simulink model "ASLquad_onboardRobustMPC_mdl"  (Simulink 8.1)
settings: Solver=ode45  StartTime=0.0  StopTime=10.0  RelTol=1e-3
values from neighbouring files (symbols this model uses):
  ASLquad_RobustMPC =     [ASLquad_RobustMPC_v2x.mat]    (also in ASLquad_RobustMPC_v3_x_Nfour.mat; ASLquad_RobustMPC_v3xyz.mat; ASLquad_RobustMPC_v3xyz_v2.mat; ASLquad_RobustMPC_v3xz.mat)
libraries: Robust_MPC_Library x6
settings Model: Creator=Kostas  LastModifiedBy=Kostas
settings DataIOCC: SignalLoggingSaveFormat=Dataset
settings OptimizationCC: ExpressionDepthLimit=128
settings DebuggingCC: FcnCallInpInsideContextMsg=EnableAllAsError
settings GRTTargetCC: CombineOutputUpdateFcns=on  GRTInterface=off

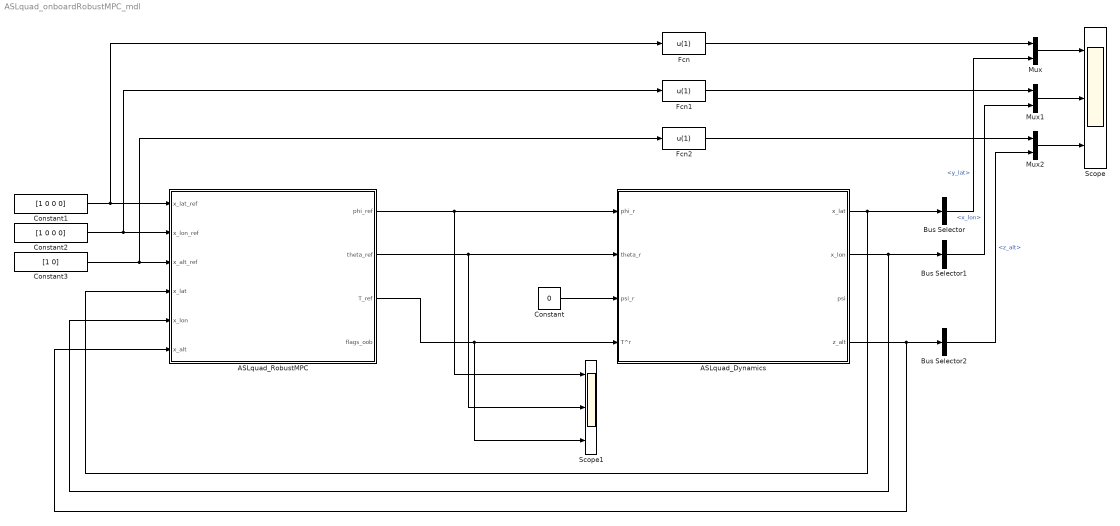
== system ASLquad_onboardRobustMPC_mdl ==
  ASLquad_Dynamics : Subsystem
  ASLquad_RobustMPC : Subsystem
  Bus Selector : BusSelector  OutputSignals=y_lat
  Bus Selector1 : BusSelector  OutputSignals=x_lon
  Bus Selector2 : BusSelector  OutputSignals=z_alt
  Constant : Constant  Value=0
  Constant1 : Constant  Value=[1 0 0 0]
  Constant2 : Constant  Value=[1 0 0 0]
  Constant3 : Constant  Value=[1 0]
  Fcn : Fcn  Expr=u(1)
  Fcn1 : Fcn  Expr=u(1)
  Fcn2 : Fcn  Expr=u(1)
  Mux : Mux  Inputs=2
  Mux1 : Mux  Inputs=2
  Mux2 : Mux  Inputs=2
  Scope : Scope  NumInputPorts=3
      settings: YMin=0.9995~-5~-5  YMax=1.00525~5~5
  Scope1 : Scope  NumInputPorts=3
      settings: YMin=-25~-5~-5  YMax=325~5~5
  wires:
  ASLquad_RobustMPC/1(phi_ref) -> Scope1/1, ASLquad_Dynamics/1(phi_r)
  ASLquad_RobustMPC/2(theta_ref) -> Scope1/2, ASLquad_Dynamics/2(theta_r)
  ASLquad_RobustMPC/3(T_ref) -> Scope1/3, ASLquad_Dynamics/4(T^r)
  Constant/1 -> ASLquad_Dynamics/3(psi_r)
  ASLquad_Dynamics/1(x_lat) -> Bus Selector/1, ASLquad_RobustMPC/4(x_lat)
  ASLquad_Dynamics/2(x_lon) -> Bus Selector1/1, ASLquad_RobustMPC/5(x_lon)
  ASLquad_Dynamics/4(z_alt) -> Bus Selector2/1, ASLquad_RobustMPC/6(x_alt)
  Constant2/1 -> Fcn1/1, ASLquad_RobustMPC/2(x_lon_ref)
  Constant3/1 -> Fcn2/1, ASLquad_RobustMPC/3(x_alt_ref)
  Constant1/1 -> Fcn/1, ASLquad_RobustMPC/1(x_lat_ref)
  Fcn/1 -> Mux/1
  Fcn1/1 -> Mux1/1
  Fcn2/1 -> Mux2/1
  Bus Selector/1 -> Mux/2  "<y_lat>"
  Bus Selector1/1 -> Mux1/2  "<x_lon>"
  Bus Selector2/1 -> Mux2/2  "<z_alt>"
  Mux/1 -> Scope/1
  Mux1/1 -> Scope/2
  Mux2/1 -> Scope/3

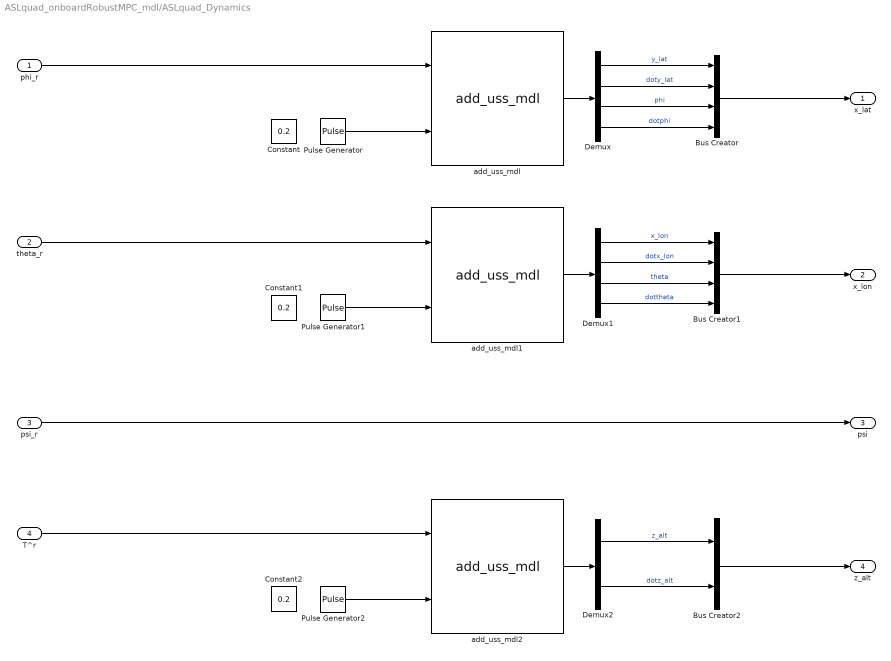
== system ASLquad_onboardRobustMPC_mdl/ASLquad_Dynamics ==
  phi_r : Inport
  theta_r : Inport  Port=2
  psi_r : Inport  Port=3
  T^r : Inport  Port=4
  Bus Creator : BusCreator
  Bus Creator1 : BusCreator
  Bus Creator2 : BusCreator  Inputs=2
  Constant : Constant  Value=0.2
  Constant1 : Constant  Value=0.2
  Constant2 : Constant  Value=0.2
  Demux : Demux
  Demux1 : Demux
  Demux2 : Demux  Outputs=2
  Pulse Generator : DiscretePulseGenerator  PulseType=Time based  Amplitude=.2  Period=2.5  PulseWidth=50
  Pulse Generator1 : DiscretePulseGenerator  PulseType=Time based  Amplitude=.2  Period=2.5  PulseWidth=50
  Pulse Generator2 : DiscretePulseGenerator  PulseType=Time based  Amplitude=.2  Period=2.5  PulseWidth=50
  add_uss_mdl : Robust_MPC_Library/add_uss_mdl  add_usys_d_struct=add_usys_y_d
  add_uss_mdl1 : Robust_MPC_Library/add_uss_mdl  add_usys_d_struct=add_usys_x_d
  add_uss_mdl2 : Robust_MPC_Library/add_uss_mdl  add_usys_d_struct=add_usys_z_d
  x_lat : Outport
  x_lon : Outport  Port=2
  psi : Outport  Port=3
  z_alt : Outport  Port=4
  wires:
  phi_r/1 -> add_uss_mdl/1
  theta_r/1 -> add_uss_mdl1/1
  T^r/1 -> add_uss_mdl2/1
  psi_r/1 -> psi/1
  add_uss_mdl/1 -> Demux/1
  Demux/1 -> Bus Creator/1  "y_lat"
  Demux/2 -> Bus Creator/2  "doty_lat"
  Demux/3 -> Bus Creator/3  "phi"
  Demux/4 -> Bus Creator/4  "dotphi"
  Bus Creator/1 -> x_lat/1
  add_uss_mdl1/1 -> Demux1/1
  Demux1/1 -> Bus Creator1/1  "x_lon"
  Demux1/2 -> Bus Creator1/2  "dotx_lon"
  Demux1/3 -> Bus Creator1/3  "theta"
  Demux1/4 -> Bus Creator1/4  "dottheta"
  Bus Creator1/1 -> x_lon/1
  add_uss_mdl2/1 -> Demux2/1
  Demux2/1 -> Bus Creator2/1  "z_alt"
  Demux2/2 -> Bus Creator2/2  "dotz_alt"
  Bus Creator2/1 -> z_alt/1
  Pulse Generator/1 -> add_uss_mdl/2
  Pulse Generator1/1 -> add_uss_mdl1/2
  Pulse Generator2/1 -> add_uss_mdl2/2

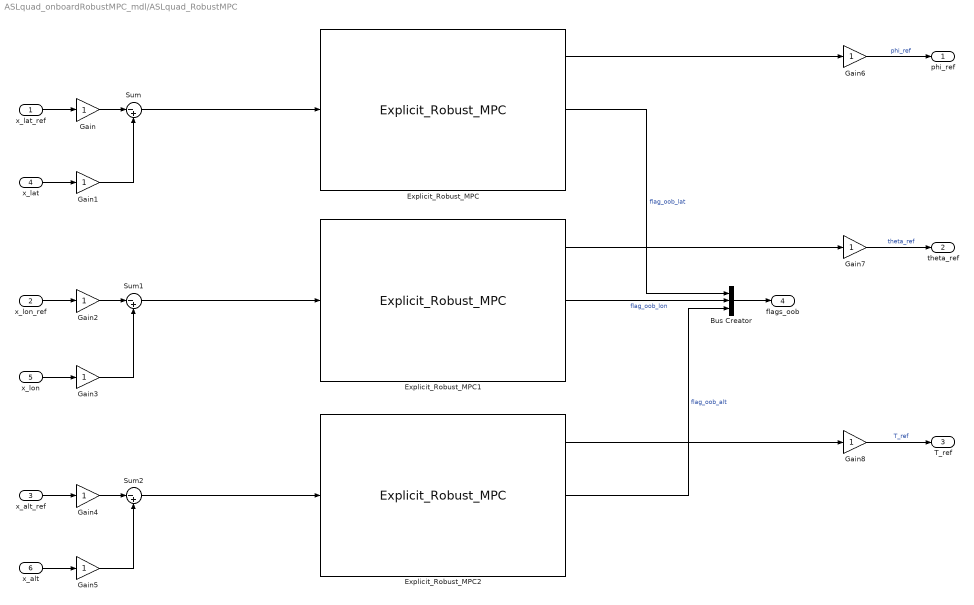
== system ASLquad_onboardRobustMPC_mdl/ASLquad_RobustMPC ==
  x_lat_ref : Inport
  x_lon_ref : Inport  Port=2
  x_alt_ref : Inport  Port=3
  x_lat : Inport  Port=4
  x_lon : Inport  Port=5
  x_alt : Inport  Port=6
  Bus Creator : BusCreator  Inputs=3
  Explicit_Robust_MPC : Robust_MPC_Library/Explicit_Robust_MPC  H=ASLquad_RobustMPC.Ydir.H  K=ASLquad_RobustMPC.Ydir.K  F=ASLquad_RobustMPC.Ydir.F  G=ASLquad_RobustMPC.Ydir.G  Nc=ASLquad_RobustMPC.Ydir.Nc  Nx=ASLquad_RobustMPC.Ydir.Nx  Hi_init=zeros(100,ASLquad_RobustMPC.Ydir.Nx)  Ki_init=zeros(100,ASLquad_RobustMPC.Ydir.Nu)
  Explicit_Robust_MPC1 : Robust_MPC_Library/Explicit_Robust_MPC  H=ASLquad_RobustMPC.Xdir.H  K=ASLquad_RobustMPC.Xdir.K  F=ASLquad_RobustMPC.Xdir.F  G=ASLquad_RobustMPC.Xdir.G  Nc=ASLquad_RobustMPC.Xdir.Nc  Nx=ASLquad_RobustMPC.Xdir.Nx  Hi_init=zeros(100,ASLquad_RobustMPC.Xdir.Nx)  Ki_init=zeros(100,ASLquad_RobustMPC.Xdir.Nu)
  Explicit_Robust_MPC2 : Robust_MPC_Library/Explicit_Robust_MPC  H=ASLquad_RobustMPC.Zdir.H  K=ASLquad_RobustMPC.Zdir.K  F=ASLquad_RobustMPC.Zdir.F  G=ASLquad_RobustMPC.Zdir.G  Nc=ASLquad_RobustMPC.Zdir.Nc  Nx=ASLquad_RobustMPC.Zdir.Nx  Hi_init=zeros(100,ASLquad_RobustMPC.Zdir.Nx)  Ki_init=zeros(100,ASLquad_RobustMPC.Zdir.Nu)
  Gain : Gain  SampleTime=ASLquad_RobustMPC.Ydir.Ts
  Gain1 : Gain  SampleTime=ASLquad_RobustMPC.Ydir.Ts
  Gain2 : Gain  SampleTime=ASLquad_RobustMPC.Xdir.Ts
  Gain3 : Gain  SampleTime=ASLquad_RobustMPC.Xdir.Ts
  Gain4 : Gain  SampleTime=ASLquad_RobustMPC.Zdir.Ts
  Gain5 : Gain  SampleTime=ASLquad_RobustMPC.Zdir.Ts
  Gain6 : Gain  SampleTime=ASLquad_RobustMPC.Ydir.Ts
  Gain7 : Gain  SampleTime=ASLquad_RobustMPC.Xdir.Ts
  Gain8 : Gain  SampleTime=ASLquad_RobustMPC.Zdir.Ts
  Sum : Sum  Inputs=|-+
  Sum1 : Sum  Inputs=|-+
  Sum2 : Sum  Inputs=|-+
  phi_ref : Outport
  theta_ref : Outport  Port=2
  T_ref : Outport  Port=3
  flags_oob : Outport  Port=4
  wires:
  x_lat_ref/1 -> Gain/1
  x_lat/1 -> Gain1/1
  x_lon_ref/1 -> Gain2/1
  x_lon/1 -> Gain3/1
  x_alt_ref/1 -> Gain4/1
  x_alt/1 -> Gain5/1
  Sum1/1 -> Explicit_Robust_MPC1/1
  Sum2/1 -> Explicit_Robust_MPC2/1
  Explicit_Robust_MPC1/1 -> Gain7/1
  Explicit_Robust_MPC2/1 -> Gain8/1
  Explicit_Robust_MPC/2 -> Bus Creator/1  "flag_oob_lat"
  Explicit_Robust_MPC1/2 -> Bus Creator/2  "flag_oob_lon"
  Explicit_Robust_MPC2/2 -> Bus Creator/3  "flag_oob_alt"
  Bus Creator/1 -> flags_oob/1
  Gain/1 -> Sum/1
  Gain1/1 -> Sum/2
  Gain2/1 -> Sum1/1
  Gain3/1 -> Sum1/2
  Gain4/1 -> Sum2/1
  Gain5/1 -> Sum2/2
  Gain6/1 -> phi_ref/1  "phi_ref"
  Gain7/1 -> theta_ref/1  "theta_ref"
  Gain8/1 -> T_ref/1  "T_ref"
  Sum/1 -> Explicit_Robust_MPC/1
  Explicit_Robust_MPC/1 -> Gain6/1
